simulink model "Lab7-P3_247-410-VA_LeonardoFusser"  (R2021a)
settings: Solver=FixedStepAuto  StartTime=0.0  StopTime=10  FixedStep=0.01  RelTol=1e-3
settings Model: Creator=Leonardo Fusser  LastModifiedBy=Leonardo Fusser

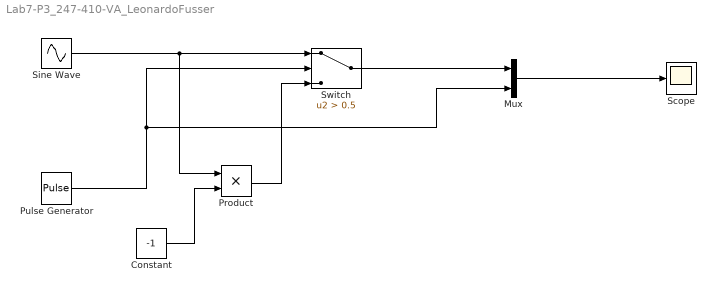
== system Lab7-P3_247-410-VA_LeonardoFusser ==
  Constant : Constant  Value=-1
  Mux : Mux  Inputs=2
  Product : Product
  Pulse Generator : DiscretePulseGenerator  PulseType=Time based  PulseWidth=50
  Scope : Scope
  Sine Wave : Sin  Frequency=2*pi*2  SampleTime=0.010
  Switch : Switch  Criteria=u2 > Threshold  Threshold=0.5
  wires:
  Mux/1 -> Scope/1
  Product/1 -> Switch/3
  Sine Wave/1 -> Product/1, Switch/1
  Pulse Generator/1 -> Mux/2, Switch/2
  Constant/1 -> Product/2
  Switch/1 -> Mux/1
